simulink model "pfb_wideband_functest"  (R2019a)
settings: Solver=VariableStepAuto  StartTime=0.0  StopTime=12000  RelTol=1e-3
values from neighbouring files (symbols this model uses):
  d0 = input_sig(1:wideband_factor:nof_points)    [filterbank_functest_input.m]    (also in pfb_functest_deinterleave_input.m = noise_sig(1:2:end); pfb_functest_script.m = sig_2(1:wideband_factor*nof_streams:nof_points); prefilter_functest_script.m; wideband_fft_functest_script.m = real_sig(1:wideband_factor:end))
  d1 = input_sig(2:wideband_factor:nof_points)    [filterbank_functest_input.m]    (also in pfb_functest_deinterleave_input.m = real_sig(1:2:end); pfb_functest_script.m = sig_1(1:wideband_factor*nof_streams:nof_points); prefilter_functest_script.m; wideband_fft_functest_script.m = noise_sig(1:wideband_factor:end))
  d2 = noise_sig(2:2:end)    [pfb_functest_deinterleave_input.m]    (also in pfb_functest_script.m = sig_2(2:wideband_factor*nof_streams:nof_points); wideband_fft_functest_script.m = real_sig(2:wideband_factor:end); wideband_functest_deinterleave_input.m; wideband_slim_functest_deinterleave_input.m)
  d3 = real_sig(2:2:end)    [pfb_functest_deinterleave_input.m]    (also in pfb_functest_script.m = sig_1(2:wideband_factor*nof_streams:nof_points); wideband_fft_functest_script.m = noise_sig(2:wideband_factor:end); wideband_functest_deinterleave_input.m; wideband_slim_functest_deinterleave_input.m)
  nof_points = 128    [filterbank_functest_input.m]    (also in pfb_functest_script.m = 1024; prefilter_functest_script.m; wideband_fft_functest_script.m = 1024)
  shift_schedule = 1023    [pfb_functest_script.m]    (also in wideband_fft_functest_script.m = 0)
undefined symbols (not defined in the file or in its folder): PFB, WB_PFB
libraries: xbsIndex_r4 x46, casper_library_misc x2
settings Model: Creator=mybur  LastModifiedBy=mybur

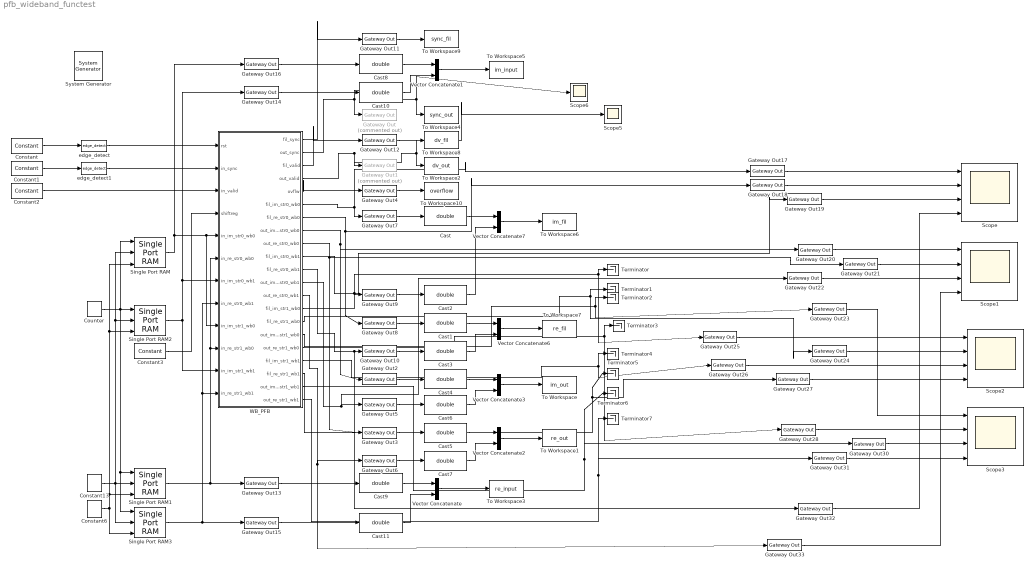
== system pfb_wideband_functest ==
  " System Generator" : xbsIndex_r4/ System Generator  Tag=genX  xilinxfamily=kintex7  part=xc7k160t  speed=-1  package=fbg484  synthesis_tool=Vivado  clock_wrapper=Clock Enables  directory=./netlist  proj_type=Vivado  Synth_file=Vivado Synthesis Defaults  Impl_file=Vivado Implementation Defaults  testbench=off  simulink_period=1  sysclk_period=10  dcm_input_clock_period=10  incr_netlist=off  trim_vbits=Everywhere in SubSystem  dbl_ovrd=According to Block Masks  core_generation=According to Block Masks  run_coregen=off  deprecated_control=off  eval_field=0  block_type=sysgen
  Cast{,1..11} (12 alike) : DataTypeConversion  OutDataTypeStr=double  RndMeth=Nearest
  Constant : xbsIndex_r4/Constant  const=1  gui_display_data_type=Boolean  arith_type=Boolean  n_bits=16  bin_pt=14  preci_type=Single  exp_width=8  frac_width=24  explicit_period=on  period=1  equ=P=C  opselect=C  inp2=PCIN>>17  opr=+  inp1=P  carry=CIN  dbl_ovrd=off  block_type=constant
  Constant1 : xbsIndex_r4/Constant  const=1  gui_display_data_type=Boolean  arith_type=Boolean  n_bits=16  bin_pt=14  preci_type=Single  exp_width=8  frac_width=24  explicit_period=on  period=1  equ=P=C  opselect=C  inp2=PCIN>>17  opr=+  inp1=P  carry=CIN  dbl_ovrd=off  block_type=constant
  Constant13 : xbsIndex_r4/Constant  const=0  gui_display_data_type=Fixed-point  arith_type=Signed (2's comp)  n_bits=input_data_width  bin_pt=0  preci_type=Single  exp_width=8  frac_width=24  explicit_period=on  period=1  equ=P=C  opselect=C  inp2=PCIN>>17  opr=+  inp1=P  carry=CIN  dbl_ovrd=off  block_type=constant
  Constant2 : xbsIndex_r4/Constant  const=1  gui_display_data_type=Boolean  arith_type=Boolean  n_bits=1  bin_pt=0  preci_type=Single  exp_width=8  frac_width=24  explicit_period=on  period=1  equ=P=C  opselect=C  inp2=PCIN>>17  opr=+  inp1=P  carry=CIN  dbl_ovrd=off  block_type=constant
  Constant3 : xbsIndex_r4/Constant  const=shift_schedule  gui_display_data_type=Fixed-point  arith_type=Unsigned  n_bits=log2(nof_points)  bin_pt=0  preci_type=Single  exp_width=8  frac_width=24  explicit_period=on  period=1  equ=P=C  opselect=C  inp2=PCIN>>17  opr=+  inp1=P  carry=CIN  dbl_ovrd=off  block_type=constant
  Constant6 : xbsIndex_r4/Constant  const=0  gui_display_data_type=Boolean  arith_type=Boolean  n_bits=1  bin_pt=0  preci_type=Single  exp_width=8  frac_width=24  explicit_period=on  period=1  equ=P=C  opselect=C  inp2=PCIN>>17  opr=+  inp1=P  carry=CIN  dbl_ovrd=off  block_type=constant
  Counter : xbsIndex_r4/Counter  cnt_type=Free Running  cnt_to=Inf  operation=Up  start_count=0  cnt_by_val=1  arith_type=Unsigned  n_bits=9  bin_pt=0  load_pin=off  rst=off  en=off  explicit_period=on  period=1  use_behavioral_HDL=off  implementation=Fabric  dbl_ovrd=off  block_type=counter
  Gateway Out : xbsIndex_r4/Gateway Out  Commented=on  inherit_from_input=on  hdl_port=on  rows=1  columns=1  UseAsDAC=off  DACChannel='1'  interface=None  automatic_assignment=on  address_offset=hex2dec('00')  intf_name=''  intf_description=''  timing_constraint=None  locs_specified=off  LOCs={}  io_standard={}  block_type=gatewayout
  Gateway Out1 : xbsIndex_r4/Gateway Out  Commented=on  inherit_from_input=off  hdl_port=off  rows=1  columns=1  UseAsDAC=off  DACChannel='1'  interface=None  automatic_assignment=on  address_offset=hex2dec('00')  intf_name=''  intf_description=''  timing_constraint=None  locs_specified=off  LOCs={}  io_standard={}  block_type=gatewayout
  Gateway Out{2..12} (11 alike) : xbsIndex_r4/Gateway Out  inherit_from_input=on  hdl_port=on  rows=1  columns=1  UseAsDAC=off  DACChannel='1'  interface=None  automatic_assignment=on  address_offset=hex2dec('00')  intf_name=''  intf_description=''  timing_constraint=None  locs_specified=off  LOCs={}  io_standard={}  block_type=gatewayout
  Gateway Out{13..16} (4 alike) : xbsIndex_r4/Gateway Out  inherit_from_input=on  hdl_port=off  rows=1  columns=1  UseAsDAC=off  DACChannel='1'  interface=None  automatic_assignment=on  address_offset=hex2dec('00')  intf_name=''  intf_description=''  timing_constraint=None  locs_specified=off  LOCs={}  io_standard={}  block_type=gatewayout
  Gateway Out{17..28,30..33} (16 alike) : xbsIndex_r4/Gateway Out  inherit_from_input=off  hdl_port=off  rows=1  columns=1  UseAsDAC=off  DACChannel='1'  interface=None  automatic_assignment=on  address_offset=hex2dec('00')  intf_name=''  intf_description=''  timing_constraint=None  locs_specified=off  LOCs={}  io_standard={}  block_type=gatewayout
  Scope{,1..3} (4 alike) : Scope  NumInputPorts=4
  Scope5 : Scope
  Scope6 : Scope
  Single Port RAM : xbsIndex_r4/Single Port RAM  depth=512  initVector=[d0]  distributed_mem=Block RAM  write_mode=Read After Write  rst=off  init_reg=0  en=off  optimize_latency=off  latency=1  optimize=Area  dbl_ovrd=off  simulation_type=fast_sim  block_type=spram
  Single Port RAM1 : xbsIndex_r4/Single Port RAM  depth=512  initVector=[d1]  distributed_mem=Block RAM  write_mode=Read After Write  rst=off  init_reg=0  en=off  optimize_latency=off  latency=1  optimize=Area  dbl_ovrd=off  simulation_type=fast_sim  block_type=spram
  Single Port RAM2 : xbsIndex_r4/Single Port RAM  depth=512  initVector=[d2]  distributed_mem=Block RAM  write_mode=Read After Write  rst=off  init_reg=0  en=off  optimize_latency=off  latency=1  optimize=Area  dbl_ovrd=off  simulation_type=fast_sim  block_type=spram
  Single Port RAM3 : xbsIndex_r4/Single Port RAM  depth=512  initVector=[d3]  distributed_mem=Block RAM  write_mode=Read After Write  rst=off  init_reg=0  en=off  optimize_latency=off  latency=1  optimize=Area  dbl_ovrd=off  simulation_type=fast_sim  block_type=spram
  Terminator{,1..7} (8 alike) : Terminator
  To Workspace : ToWorkspace  VariableName=im_out  SaveFormat=Timeseries  SampleTime=-1
  To Workspace1 : ToWorkspace  VariableName=re_out  SaveFormat=Timeseries  SampleTime=-1
  To Workspace10 : ToWorkspace  VariableName=overflow  SaveFormat=Timeseries  SampleTime=-1
  To Workspace2 : ToWorkspace  VariableName=dv_out  SaveFormat=Timeseries  SampleTime=-1
  To Workspace3 : ToWorkspace  VariableName=re_input  SaveFormat=Timeseries  SampleTime=-1
  To Workspace4 : ToWorkspace  VariableName=sync_out  SaveFormat=Timeseries  SampleTime=-1
  To Workspace5 : ToWorkspace  VariableName=im_input  SaveFormat=Timeseries  SampleTime=-1
  To Workspace6 : ToWorkspace  VariableName=im_fil  SaveFormat=Timeseries  SampleTime=-1
  To Workspace7 : ToWorkspace  VariableName=re_fil  SaveFormat=Timeseries  SampleTime=-1
  To Workspace8 : ToWorkspace  VariableName=dv_fil  SaveFormat=Timeseries  SampleTime=-1
  To Workspace9 : ToWorkspace  VariableName=sync_fil  SaveFormat=Timeseries  SampleTime=-1
  Vector Concatenate{,1..3,6..7} (6 alike) : Concatenate  NumInputs=wideband_factor
  WB_PFB : Subsystem  AncestorBlock=PFB/WB_PFB  mask(Wideband Polyphase Filterbank Block){use_separate=on, use_fft_shift=off, use_reorder=on, alt_output=off, wb_factor=2, nof_points=10, nof_taps=2, nof_wb_streams=2, nof_chan=0, xtra_dat_sigs=off, big_endian_wb_in=off, use_prefilter=on, dont_flip_channels=off, out_gain_w=0, win="hanning", fwidth=1.0, backoff_w=0, fil_in_dat_w=18, fil_out_dat_w=18, fil_coef_dat_w=18, twid_dat_w=18, fft_stage_dat_w=18, fft_out_dat_w=18, fft_guard_enable=on, fft_guard_w=2, fft_ovflw_behav="WRAP", fft_use_round=1, pipe_reo_in_place=on, use_dsp="YES", use_variant="4DSP", fft_ram_primitive="block", max_addr_w=8, fil_ram_primitive="block", vendor_technology=Xilinx}
      mask prompts: use_separate "Separate re/im outputs"; use_fft_shift "Reorder frequencies"; use_reorder "Bit reverse output"; alt_output "Alter output data stream"; wb_factor "Wideband factor"; nof_points "Number of points (2^nof_pts)"; nof_taps "Number of taps"; nof_wb_streams "Number of wideband streams"; nof_chan "Number of channels (2^nof_chan)"; xtra_dat_sigs "Extra control signals"; big_endian_wb_in "Big endian input data"; use_prefilter "Enable prefilter"; dont_flip_channels "Don't flip channels"; out_gain_w "Output gain width"; win "Window function"; backoff_w "Filter backoff width"; fil_in_dat_w "Prefilter input data width"; fil_out_dat_w "Prefilter output data width"; fil_coef_dat_w "Prefilter coefficient data width"; twid_dat_w "FFT twiddle data width"; fft_stage_dat_w "FFT stage data width"; fft_out_dat_w "FFT output data width"; fft_guard_enable "Guard FFT input data"; fft_guard_w "FFT guard data width"; fft_ovflw_behav "FFT overflow behaviour"; fft_use_round "FFT rounding mode: 0-Truncate, 1-Round Even, 2-Round Infinite"; pipe_reo_in_place "Use single pipelined FFT reorder buffer"; use_dsp "Use DSP for Cmults"; use_variant "Cmult options"; fft_ram_primitive "FFT Ram Primitive"; max_addr_w "Twiddle Max Address Width"; fil_ram_primitive "Prefilter Ram Primitive"; vendor_technology "Vendor technology"
      mask help: The Wideband Poly Phase FilterBank can process a datastream that is partly applied in serial and partly applied in parallel. It consists of a Poly Phase Filter (PPF) and a Fast Fourier Transform (FFT). It distinguishes from a single FFT by the PPF, that acts as a window function to produce a flat response across the channel, and excellent suppression of out-of-band signals.
      mask init:
      | Simulink.Block.eval([gcb, '/wb_pfb']);
      |  
      | wb_pfb_subsys2bb_knit();
      mask Help: https://casper-dspdevel.readthedocs.io/en/latest/wideband_pfb.html
      mask Callback use_separate:
      | enab = get_param(gcb,'use_separate');
      | 
      | % Set the 'MaskVisibilities' property for each parameters
      | if strcmp(enab,'on')
      |     set_param(gcb,'use_reorder','on');
      |     set_param(gcb,'use_fft_shift','off');
      |     set_param(gcb,'MaskEnables',{'on','off','off','on','on','on','on','on','on','on','on','on','on','on','on','on','on','on','on','on','on','on','on','on','on','on','on','on','on','on','on','on','on','on'});
      | else
      |     set_param(gcb,'MaskEnables',{'on','on','on','on','on','on','on','on','on','on','on','on','on','on','on','on','on','on','on','on','on','on','on','on','on','on','on','on','on','on','on','on','on','on'});
      | end
      mask Callback use_fft_shift:
      | enab = get_param(gcb,'use_fft_shift');
      | 
      | % Set the 'MaskVisibilities' property for each parameters
      | if strcmp(enab,'on')
      |     set_param(gcb,'use_reorder','on');
      |     set_param(gcb,'MaskEnables',{'on','on','off','on','on','on','on','on','on','on','on','on','on','on','on','on','on','on','on','on','on','on','on','on','on','on','on','on','on','on','on','on','on','on'});
      | else
      |     set_param(gcb,'MaskEnables',{'on','on','on','on','on','on','on','on','on','on','on','on','on','on','on','on','on','on','on','on','on','on','on','on','on','on','on','on','on','on','on','on','on','on'});
      | end
      mask TypeOptions win: "hanning" | "hamming" | "blackman"
      mask Callback fft_guard_enable:
      | enab = get_param(gcb,'fft_guard_enable');
      | 
      | % Set the 'MaskVisibilities' property for each parameters
      | if strcmp(enab,'on')
      |     set_param(gcb,'MaskVisibilities',{'on','on','on','on','on','on','on','on','on','on','on','on','on','on','on','on','on','on','on','on','on','on','on','on','on','on','on','on','on','on','on','on','on','on'});
      | else
      |     set_param(gcb,'MaskVisibilities',{'on','on','on','on','on','on','on','on','on','on','on','on','on','on','on','on','on','on','on','on','on','on','on','on','off','on','on','on','on','on','on','on','on','on'});
      | end
      mask TypeOptions fft_ovflw_behav: "SATURATE" | "WRAP"
      mask TypeOptions fft_use_round: 0 | 1 | 2
      mask TypeOptions use_dsp: "YES" | "NO"
      mask TypeOptions use_variant: "4DSP" | "3DSP"
      mask TypeOptions fft_ram_primitive: "block" | "distributed" | "ultra" | "auto"
      mask TypeOptions fil_ram_primitive: "block" | "distributed" | "ultra" | "auto"
      mask TypeOptions vendor_technology: Xilinx | UniBoard
      mask DialogControl DescTextVar Prompt: The wpfb unit is a Wideband Poly Phase FilterBank which can process a datastream that is partly applied in serial and partly applied in parallel. It consists of a Poly Phase Filter (PPF) and a Fast Fourier Transform (FFT). The wpfb distinguishes from a single FFT by the PPF that functions as a window function in order to produce a flat response across the channel, but also provides excellent suppression of out-of-band signals. https://casper-dspdevel.readthedocs.io/en/latest/wideband_pfb.html
      mask DialogControl pfb_params Prompt: PFB Parameters
      mask DialogControl pfb Prompt: PFB
      mask DialogControl filter Prompt: FILTER
      mask DialogControl fft Prompt: FFT
      mask DialogControl synth Prompt: SYNTH/IMP
  edge_detect : casper_library_misc/edge_detect  edge=Rising  polarity=Active High  x_in=[0 0.08 0.08 0.16 0.16 0.24 0.24 0.32 0.32 0.4]  y_in="[-1 -1  1  1  1  1  1  1  1  1]"  x_out=[0.6 0.68 0.68 0.76 0.76 0.84 0.84 0.92 0.92 1]  y_out="[-1 -1  1  1 -1 -1 -1 -1 -1 -1]"
  edge_detect1 : casper_library_misc/edge_detect  edge=Rising  polarity=Active High  x_in=[0 0.08 0.08 0.16 0.16 0.24 0.24 0.32 0.32 0.4]  y_in="[-1 -1  1  1  1  1  1  1  1  1]"  x_out=[0.6 0.68 0.68 0.76 0.76 0.84 0.84 0.92 0.92 1]  y_out="[-1 -1  1  1 -1 -1 -1 -1 -1 -1]"
  wires:
  WB_PFB/8(out_im_str0_wb0) -> Gateway Out2/1, Gateway Out20/1
  WB_PFB/9(out_re_str0_wb0) -> Gateway Out3/1, Gateway Out21/1
  Vector Concatenate1/1 -> To Workspace5/1
  WB_PFB/12(out_im_str0_wb1) -> Gateway Out5/1, Gateway Out22/1
  Gateway Out3/1 -> Cast5/1
  Gateway Out7/1 -> Cast/1
  Gateway Out10/1 -> Cast3/1
  Gateway Out14/1 -> Cast10/1
  Gateway Out2/1 -> Cast4/1
  Gateway Out6/1 -> Cast7/1
  Gateway Out13/1 -> Cast9/1
  Gateway Out11/1 -> To Workspace9/1
  Gateway Out15/1 -> Cast11/1
  Gateway Out4/1 -> To Workspace10/1
  Cast8/1 -> Vector Concatenate1/1
  Vector Concatenate2/1 -> To Workspace1/1
  Cast9/1 -> Vector Concatenate/1
  Cast10/1 -> Vector Concatenate1/2
  Cast11/1 -> Vector Concatenate/2
  Gateway Out12/1 -> To Workspace8/1
  WB_PFB/13(out_re_str0_wb1) -> Gateway Out6/1, Gateway Out33/1
  Gateway Out5/1 -> Cast6/1
  Gateway Out16/1 -> Cast8/1
  Cast6/1 -> Vector Concatenate3/2
  Cast7/1 -> Vector Concatenate2/2
  Constant1/1 -> edge_detect1/1
  Cast5/1 -> Vector Concatenate2/1
  Vector Concatenate/1 -> To Workspace3/1
  Cast4/1 -> Vector Concatenate3/1
  Constant6/1 -> Single Port RAM2/3, Single Port RAM/3, Single Port RAM1/3, Single Port RAM3/3
  Cast3/1 -> Vector Concatenate6/2
  Constant2/1 -> WB_PFB/3(in_valid)
  Cast2/1 -> Vector Concatenate7/2
  Cast1/1 -> Vector Concatenate6/1
  Constant/1 -> edge_detect/1
  WB_PFB/5(ovflw) -> Gateway Out4/1
  Cast/1 -> Vector Concatenate7/1
  Gateway Out9/1 -> Cast2/1
  WB_PFB/11(fil_re_str0_wb1) -> Gateway Out32/1, Gateway Out10/1
  WB_PFB/7(fil_re_str0_wb0) -> Gateway Out18/1, Gateway Out8/1
  WB_PFB/6(fil_im_str0_wb0) -> Gateway Out17/1, Gateway Out7/1
  edge_detect1/1 -> WB_PFB/2(in_sync)
  Constant13/1 -> Single Port RAM2/2, Single Port RAM/2, Single Port RAM3/2, Single Port RAM1/2
  Vector Concatenate6/1 -> To Workspace7/1
  WB_PFB/2(out_sync) -> Scope6/1, To Workspace4/1, Gateway Out/1
  WB_PFB/1(fil_sync) -> Gateway Out11/1
  Single Port RAM3/1 -> WB_PFB/12(in_re_str1_wb1), WB_PFB/8(in_re_str0_wb1), Gateway Out15/1
  Single Port RAM1/1 -> WB_PFB/10(in_re_str1_wb0), WB_PFB/6(in_re_str0_wb0), Gateway Out13/1
  Gateway Out8/1 -> Cast1/1
  Vector Concatenate7/1 -> To Workspace6/1
  Vector Concatenate3/1 -> To Workspace/1
  Constant3/1 -> WB_PFB/4(shiftreg)
  Single Port RAM/1 -> WB_PFB/5(in_im_str0_wb0), WB_PFB/9(in_im_str1_wb0), Gateway Out16/1
  Counter/1 -> Single Port RAM3/1, Single Port RAM1/1, Single Port RAM2/1, Single Port RAM/1
  WB_PFB/10(fil_im_str0_wb1) -> Gateway Out19/1, Gateway Out9/1
  WB_PFB/3(fil_valid) -> Gateway Out12/1
  WB_PFB/4(out_valid) -> Scope5/1, To Workspace2/1, Gateway Out1/1
  Single Port RAM2/1 -> WB_PFB/11(in_im_str1_wb1), WB_PFB/7(in_im_str0_wb1), Gateway Out14/1
  WB_PFB/14(fil_im_str1_wb0) -> Gateway Out25/1, Terminator/1
  WB_PFB/15(fil_re_str1_wb0) -> Terminator1/1, Gateway Out24/1
  WB_PFB/16(out_im_str1_wb0) -> Terminator2/1, Gateway Out23/1
  WB_PFB/17(out_re_str1_wb0) -> Gateway Out28/1, Terminator3/1
  WB_PFB/18(fil_im_str1_wb1) -> Gateway Out26/1, Terminator4/1
  WB_PFB/19(fil_re_str1_wb1) -> Terminator5/1, Gateway Out27/1
  WB_PFB/20(out_im_str1_wb1) -> Gateway Out30/1, Terminator6/1
  WB_PFB/21(out_re_str1_wb1) -> Gateway Out31/1, Terminator7/1
  Gateway Out17/1 -> Scope/1
  Gateway Out18/1 -> Scope/2
  Gateway Out19/1 -> Scope/3
  Gateway Out20/1 -> Scope1/1
  Gateway Out21/1 -> Scope1/2
  Gateway Out22/1 -> Scope1/3
  Gateway Out24/1 -> Scope2/2
  Gateway Out25/1 -> Scope2/1
  Gateway Out26/1 -> Scope2/3
  Gateway Out27/1 -> Scope2/4
  Gateway Out28/1 -> Scope3/2
  Gateway Out23/1 -> Scope3/1
  Gateway Out30/1 -> Scope3/3
  Gateway Out31/1 -> Scope3/4
  Gateway Out32/1 -> Scope/4
  Gateway Out33/1 -> Scope1/4
  edge_detect/1 -> WB_PFB/1(rst)

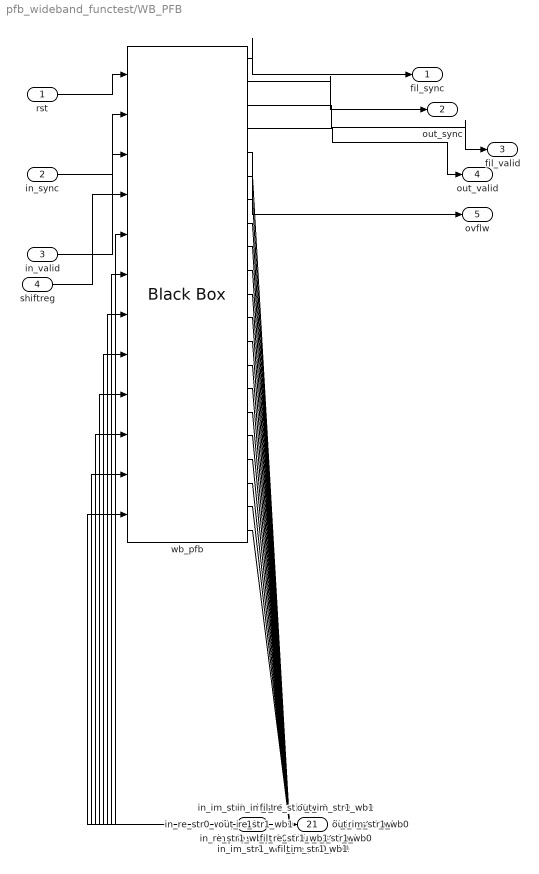
== system pfb_wideband_functest/WB_PFB ==
  rst : Inport
  in_sync : Inport  Port=2
  in_valid : Inport  Port=3
  shiftreg : Inport  Port=4
  in_im_str0_wb0 : Inport  Port=5
  in_re_str0_wb0 : Inport  Port=6
  in_im_str0_wb1 : Inport  Port=7
  in_re_str0_wb1 : Inport  Port=8
  in_im_str1_wb0 : Inport  Port=9
  in_re_str1_wb0 : Inport  Port=10
  in_im_str1_wb1 : Inport  Port=11
  in_re_str1_wb1 : Inport  Port=12
  wb_pfb : xbsIndex_r4/Black Box  init_code=wbpfb_unit_top_config  sim_method=ISE Simulator  verbose=off  block_type=blackbox2
  fil_sync : Outport
  out_sync : Outport  Port=2
  fil_valid : Outport  Port=3
  out_valid : Outport  Port=4
  ovflw : Outport  Port=5
  fil_im_str0_wb0 : Outport  Port=6
  fil_re_str0_wb0 : Outport  Port=7
  out_im_str0_wb0 : Outport  Port=8
  out_re_str0_wb0 : Outport  Port=9
  fil_im_str0_wb1 : Outport  Port=10
  fil_re_str0_wb1 : Outport  Port=11
  out_im_str0_wb1 : Outport  Port=12
  out_re_str0_wb1 : Outport  Port=13
  fil_im_str1_wb0 : Outport  Port=14
  fil_re_str1_wb0 : Outport  Port=15
  out_im_str1_wb0 : Outport  Port=16
  out_re_str1_wb0 : Outport  Port=17
  fil_im_str1_wb1 : Outport  Port=18
  fil_re_str1_wb1 : Outport  Port=19
  out_im_str1_wb1 : Outport  Port=20
  out_re_str1_wb1 : Outport  Port=21
  wires:
  rst/1 -> wb_pfb/1
  in_sync/1 -> wb_pfb/2
  in_valid/1 -> wb_pfb/3
  shiftreg/1 -> wb_pfb/4
  wb_pfb/1 -> fil_sync/1
  wb_pfb/2 -> out_sync/1
  wb_pfb/3 -> fil_valid/1
  wb_pfb/4 -> out_valid/1
  wb_pfb/5 -> ovflw/1
  in_im_str0_wb0/1 -> wb_pfb/5
  in_re_str0_wb0/1 -> wb_pfb/6
  wb_pfb/6 -> fil_im_str0_wb0/1
  wb_pfb/7 -> fil_re_str0_wb0/1
  wb_pfb/14 -> out_im_str0_wb0/1
  wb_pfb/15 -> out_re_str0_wb0/1
  in_im_str0_wb1/1 -> wb_pfb/7
  in_re_str0_wb1/1 -> wb_pfb/8
  wb_pfb/8 -> fil_im_str0_wb1/1
  wb_pfb/9 -> fil_re_str0_wb1/1
  wb_pfb/16 -> out_im_str0_wb1/1
  wb_pfb/17 -> out_re_str0_wb1/1
  in_im_str1_wb0/1 -> wb_pfb/9
  in_re_str1_wb0/1 -> wb_pfb/10
  wb_pfb/10 -> fil_im_str1_wb0/1
  wb_pfb/11 -> fil_re_str1_wb0/1
  wb_pfb/18 -> out_im_str1_wb0/1
  wb_pfb/19 -> out_re_str1_wb0/1
  in_im_str1_wb1/1 -> wb_pfb/11
  in_re_str1_wb1/1 -> wb_pfb/12
  wb_pfb/12 -> fil_im_str1_wb1/1
  wb_pfb/13 -> fil_re_str1_wb1/1
  wb_pfb/20 -> out_im_str1_wb1/1
  wb_pfb/21 -> out_re_str1_wb1/1
